simulink model "Extended_model_st"  (Simulink 7.4)
settings: Solver=ode45  StartTime=0.0  StopTime=10.0  RelTol=1e-3
values from neighbouring files (symbols this model uses):
  Ask = [0 1 0 0 ... (first row only)    [H_inf_ctrl (1).m]    (also in T8_T9_T10_T11.m; pitch (1).m)
  Bsk = [0 0 0 0 ... (first row only)    [H_inf_ctrl (1).m]    (also in T8_T9_T10_T11.m; pitch (1).m)
  Csk = [0 1 0 0 ... (first row only)    [H_inf_ctrl (1).m]    (also in T8_T9_T10_T11.m; pitch (1).m)
  Dsk = zeros(2,4)    [H_inf_ctrl (1).m]    (also in T8_T9_T10_T11.m; pitch (1).m)
libraries: cstblocks x4
settings Model: Creator=Alireza  LastModifiedBy=Alireza

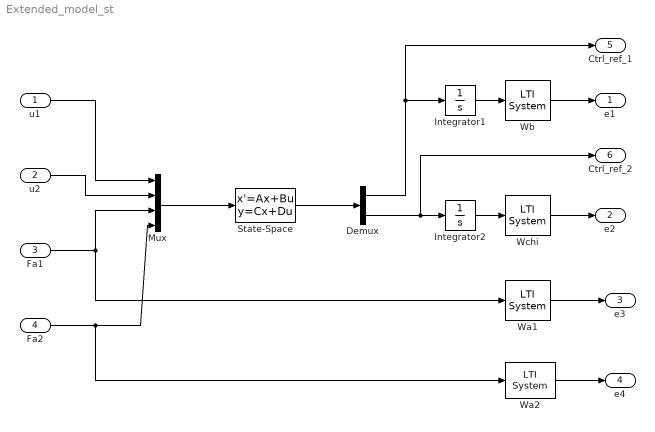
== system Extended_model_st ==
  u1 : Inport  OutDataType=fixdt(1, 16)  OutScaling=2^0
  u2 : Inport  Port=2  OutDataType=fixdt(1, 16)  OutScaling=2^0
  Fa1 : Inport  Port=3  OutDataType=fixdt(1, 16)  OutScaling=2^0
  Fa2 : Inport  Port=4  OutDataType=fixdt(1, 16)  OutScaling=2^0
  Demux : Demux  Outputs=2
  Integrator1 : Integrator
  Integrator2 : Integrator
  Mux : Mux
  State-Space : StateSpace  A=Ask  B=Bsk  C=Csk  D=Dsk
  Wa1 : cstblocks/LTI System  SystemSampleTime=-1  sys=Wa1  IC=[]
  Wa2 : cstblocks/LTI System  SystemSampleTime=-1  sys=Wa2  IC=[]
  Wb : cstblocks/LTI System  SystemSampleTime=-1  sys=Wb  IC=[]
  Wchi : cstblocks/LTI System  SystemSampleTime=-1  sys=Wchi  IC=[]
  e1 : Outport  OutDataType=fixdt(1, 16)  OutScaling=2^0
  e2 : Outport  Port=2  OutDataType=fixdt(1, 16)  OutScaling=2^0
  e3 : Outport  Port=3  OutDataType=fixdt(1, 16)  OutScaling=2^0
  e4 : Outport  Port=4  OutDataType=fixdt(1, 16)  OutScaling=2^0
  Ctrl_ref_1 : Outport  Port=5  OutDataType=fixdt(1, 16)  OutScaling=2^0
  Ctrl_ref_2 : Outport  Port=6  OutDataType=fixdt(1, 16)  OutScaling=2^0
  wires:
  u1/1 -> Mux/1
  u2/1 -> Mux/2
  Fa1/1 -> Mux/3, Wa1/1
  Fa2/1 -> Mux/4, Wa2/1
  Wa1/1 -> e3/1
  Wa2/1 -> e4/1
  Mux/1 -> State-Space/1
  State-Space/1 -> Demux/1
  Demux/1 -> Ctrl_ref_1/1, Integrator1/1
  Demux/2 -> Ctrl_ref_2/1, Integrator2/1
  Wb/1 -> e1/1
  Wchi/1 -> e2/1
  Integrator1/1 -> Wb/1
  Integrator2/1 -> Wchi/1
